simulink model "P5p5cx"  (R2017b)
settings: Solver=ode45  StartTime=0.0  StopTime=5000  RelTol=1e-3  EnableMultiTasking=on
values from neighbouring files (symbols this model uses):
  K_pd = 0.816058507166699    (= 0.816058507167)    [P5p5c.m]    (also in P5p5c_init.m)
  psi_ref = 30    [P5p5c.m]    (also in P5p5c_init.m)
  T = 70.55    [P5p5a.m]    (also in P5p5a_init.m; P5p5c.m; P5p5c_init.m; p5p1.m)
  T_f = 8.395449999999999    (= 8.39545)    [P5p5c.m]    (also in P5p5c_init.m)
libraries: simulink x2
settings Model: Creator=markh  LastModifiedBy=sondrefyhn
settings DataIOCC: LimitDataPoints=on  SaveFormat=Array  SignalLoggingSaveFormat=ModelDataLogs  SignalLoggingName=sigsOut
settings OptimizationCC: InitFltsAndDblsToZero=on  LifeSpan=inf
settings DebuggingCC: SaveWithParameterizedLinksMsg=none  UnderspecifiedInitializationDetection=Classic  MergeDetectMultiDrivingBlocksExec=none  SignalResolutionControl=TryResolveAllWithWarning  MultiTaskDSMMsg=warning  MultiTaskCondExecSysMsg=none  FcnCallInpInsideContextMsg=warning  StateNameClashWarn=warning  StrictBusMsg=None  SFUnexpectedBacktrackingDiag=warning  SFNoUnconditionalDefaultTransitionDiag=warning  SFExecutionAtInitializationDiag=none
settings HardwareCC: ProdBitPerPointer=32  ProdBitPerSizeT=32  ProdBitPerPtrDiffT=32  ProdLargestAtomicFloat=None  ProdIntDivRoundTo=Undefined  ProdEndianess=Unspecified  ProdWordSize=32  ProdHWDeviceType=32-bit Generic  TargetUnknown=on
settings ModelReferenceCC: PropagateSignalLabelsOutOfModel=off
settings RTWCC: Description=Generic Real-Time Target
settings CodeAppCC: StateflowObjectComments=on
settings GRTTargetCC: TargetFcnLib=ansi_tfl_tmw.mat  TargetLangStandard=C89/C90 (ANSI)  GeneratePreprocessorConditionals=Disable all  CombineOutputUpdateFcns=off  GRTInterface=on
settings ConfigComp: CovMetricSettings=dw  CovHtmlReporting=on  CovSaveCumulativeToWorkspaceVar=on  CovSaveSingleToWorkspaceVar=on  CovExternalEMLEnable=off

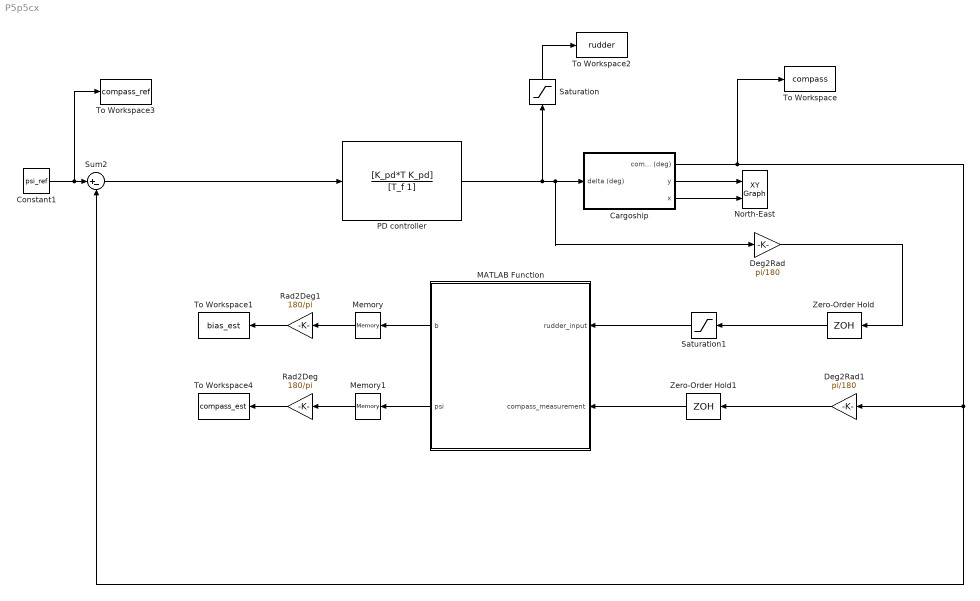
== system P5p5cx ==
  Cargoship : Subsystem  mask(Simple shipmodel for a cargo ship){noise=on, current=off, logic=off}
      mask prompts: noise "measurement noise"; logic "waves"
      mask help:
      | Measurement noise:
      | 	checked = noise on
      | 	unchecked = noise off
      |
      | Current:
      | 	checked = current on
      | 	unchecked = current off
      |
      | Waves:
      | 	checked = waves on
      | 	unchecked = waves off
      |
      | Author: Jørgen Spjøtvold, 9/10-2003
      | TTK 4115 Linear system theory.
      | Modified by Jostein Bakkeheim 26/10-2006
  Constant1 : Constant  Value=psi_ref
  Deg2Rad : Gain  Gain=pi/180
  Deg2Rad1 : Gain  Gain=pi/180
  MATLAB Function : MATLAB Function  TreatAsAtomicUnit=on
  Memory : Memory
  Memory1 : Memory
  North-East : simulink/Sinks/XY Graph  xmin=-5000  xmax=7500  ymin=-5000  ymax=5000  st=-1
  PD controller : TransferFcn  Numerator=[K_pd*T K_pd]  Denominator=[T_f 1]
  Rad2Deg : Gain  Gain=180/pi
  Rad2Deg1 : Gain  Gain=180/pi
  Saturation : Saturate  UpperLimit=45  LowerLimit=-45
  Saturation1 : Saturate  UpperLimit=45  LowerLimit=-45
  Sum2 : Sum  Inputs=|+-
  To Workspace : ToWorkspace  VariableName=compass  SaveFormat=Structure With Time  SampleTime=-1
      settings: MaxDataPoints=9999999
  To Workspace1 : ToWorkspace  VariableName=bias_est  SaveFormat=Structure With Time  SampleTime=-1
      settings: MaxDataPoints=9999999
  To Workspace2 : ToWorkspace  VariableName=rudder  SaveFormat=Structure With Time  SampleTime=-1
      settings: MaxDataPoints=9999999
  To Workspace3 : ToWorkspace  VariableName=compass_ref  SaveFormat=Structure With Time  SampleTime=-1
      settings: MaxDataPoints=9999999
  To Workspace4 : ToWorkspace  VariableName=compass_est  SaveFormat=Structure With Time  SampleTime=-1
      settings: MaxDataPoints=9999999
  Zero-Order Hold : ZeroOrderHold  SampleTime=1/10
  Zero-Order Hold1 : ZeroOrderHold  SampleTime=1/10
  wires:
  Cargoship/3(x) -> North-East/2
  Cargoship/2(y) -> North-East/1
  Constant1/1 -> To Workspace3/1, Sum2/1
  Sum2/1 -> PD controller/1
  Saturation/1 -> To Workspace2/1
  Cargoship/1(compass (deg)) -> To Workspace/1, Deg2Rad1/1, Sum2/2
  Zero-Order Hold/1 -> Saturation1/1
  Zero-Order Hold1/1 -> MATLAB Function/2(compass_measurement)
  MATLAB Function/2(psi) -> Memory1/1
  MATLAB Function/1(b) -> Memory/1
  Rad2Deg1/1 -> To Workspace1/1
  Saturation1/1 -> MATLAB Function/1(rudder_input)
  PD controller/1 -> Deg2Rad/1, Cargoship/1(delta (deg)), Saturation/1
  Deg2Rad/1 -> Zero-Order Hold/1
  Deg2Rad1/1 -> Zero-Order Hold1/1
  Rad2Deg/1 -> To Workspace4/1
  Memory1/1 -> Rad2Deg/1
  Memory/1 -> Rad2Deg1/1

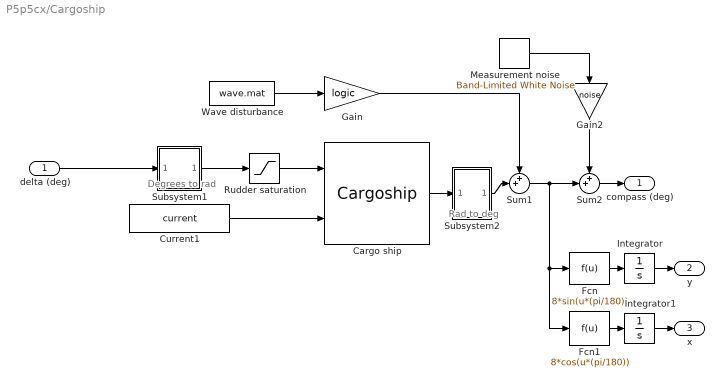
== system P5p5cx/Cargoship ==
  note: Degrees to rad
  note: Rad to deg
  delta (deg) : Inport
  Cargo ship : S-Function  FunctionName=Cargoship  SFunctionDeploymentMode=off  EnableBusSupport=off  mask(Cargo ship){}
      mask help:
      | S-function which simulates a cargo ship.
      |
      | Author: Jørgen Spjøtvold
      | 20.10-2003
      | Modified by Jostein Bakkeheim 27.10.2006
  Current1 : Constant  Value=current
  Fcn : Fcn  Expr=8*sin(u*(pi/180))
  Fcn1 : Fcn  Expr=8*cos(u*(pi/180))
  Gain : Gain  Gain=logic  SaturateOnIntegerOverflow=on  OutDataTypeStr=Inherit: Same as input  ParamDataTypeStr=Inherit: Same as input
  Gain2 : Gain  Gain=noise  SaturateOnIntegerOverflow=on  OutDataTypeStr=Inherit: Same as input  ParamDataTypeStr=Inherit: Same as input
  Integrator : Integrator
  Integrator1 : Integrator
  Measurement noise : simulink/Sources/Band-Limited White Noise  Cov=[0.001]  Ts=.5  seed=[23341]
  Rudder saturation : Saturate  UpperLimit=45*(pi/180)  LowerLimit=-45*(pi/180)
  Subsystem1 : Subsystem  mask(degrees to radians){}
      mask help: Converts degrees to radians
      mask Display: fprintf('D2R');
  Subsystem2 : Subsystem  mask(radians to degrees){}
      mask help: Converts radians to degrees
      mask Display: fprintf('R2D');
  Sum1 : Sum  Inputs=++|  SaturateOnIntegerOverflow=on
  Sum2 : Sum  Inputs=++|  SaturateOnIntegerOverflow=on
  Wave disturbance : FromFile  FileName=wave.mat  SampleTime=0
  compass (deg) : Outport
  y : Outport  Port=2
  x : Outport  Port=3
  wires:
  delta (deg)/1 -> Subsystem1/1(In1)
  Fcn/1 -> Integrator/1
  Integrator/1 -> y/1
  Fcn1/1 -> Integrator1/1
  Integrator1/1 -> x/1
  Wave disturbance/1 -> Gain/1
  Subsystem2/1(Out1) -> Sum1/2
  Gain/1 -> Sum1/1
  Sum1/1 -> Fcn/1, Fcn1/1, Sum2/2
  Cargo ship/1 -> Subsystem2/1(In1)
  Subsystem1/1(Out1) -> Rudder saturation/1
  Rudder saturation/1 -> Cargo ship/1
  Sum2/1 -> compass (deg)/1
  Measurement noise/1 -> Gain2/1
  Gain2/1 -> Sum2/1
  Current1/1 -> Cargo ship/2

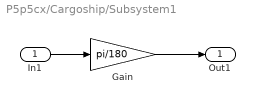
== system P5p5cx/Cargoship/Subsystem1 ==
  In1 : Inport
  Gain : Gain  Gain=pi/180  SaturateOnIntegerOverflow=on  OutDataTypeStr=Inherit: Same as input  ParamDataTypeStr=Inherit: Same as input
  Out1 : Outport
  wires:
  Gain/1 -> Out1/1
  In1/1 -> Gain/1

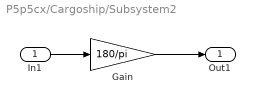
== system P5p5cx/Cargoship/Subsystem2 ==
  In1 : Inport
  Gain : Gain  Gain=180/pi  SaturateOnIntegerOverflow=on  OutDataTypeStr=Inherit: Same as input  ParamDataTypeStr=Inherit: Same as input
  Out1 : Outport
  wires:
  Gain/1 -> Out1/1
  In1/1 -> Gain/1

== matlab function P5p5cx/MATLAB Function ==
  data: rudder_input input; b output; compass_measurement input; psi output; data parameter

function [b,psi] = Kalman_filter(rudder_input,compass_measurement, data)
%%%%%%%%%%%%%%ALGORITHM FOR COMPUTING KALMAN FILTER%%%%%%%%%%%%%%%%%%%%%%%

%%Defining init flag
persistent init_flag ad bd Cd ed Q_k R prior_P_covar prior_x_est I
%%Defining the needed starting conditions
if isempty(init_flag)
    [ad, bd, Cd, ed, Q_k, R, prior_P_covar, prior_x_est, I] = deal(data.ad, data.bd, data.Cd, data.ed, data.Q_k, data.R, data.prior_P_covar, data.prior_x_est, data.I);
    init_flag = 1;
end


%%Computing Kalman gain
L_k = prior_P_covar * transpose(Cd) * (Cd * prior_P_covar * transpose(Cd) + R)^(-1);

%%Updating estimate with measurement y_k
x_est = prior_x_est + L_k * (compass_measurement - Cd * prior_x_est);

%%Computing error covariance for updated estimate
P_k = (I - L_k * Cd) * prior_P_covar * transpose(I - L_k * Cd) + L_k * R * transpose(L_k);

%%Project ahead
prior_x_est = ad * x_est + bd * rudder_input;
prior_P_covar = ad * P_k * transpose(ad) + ed * Q_k * transpose(ed);

%%Outputs
psi = x_est(3);
b = x_est(5);
end
